simulink model "zaj2simulink"  (R2020b)
settings: Solver=VariableStepAuto  StartTime=0.0  StopTime=100  RelTol=1e-3
settings Model: Creator=bilin  LastModifiedBy=bilin

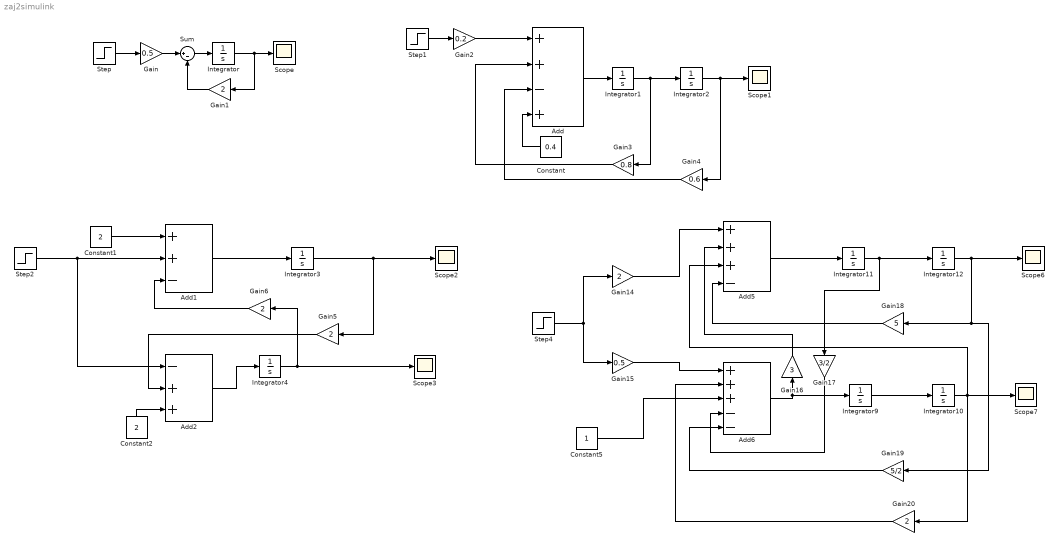
== system zaj2simulink ==
  Add : Sum  Inputs=++-+
  Add1 : Sum  Inputs=++-
  Add2 : Sum  Inputs=-++
  Add5 : Sum  Inputs=+++-
  Add6 : Sum  Inputs=+++--
  Constant : Constant  Value=0.4
  Constant1 : Constant  Value=2
  Constant2 : Constant  Value=2
  Constant5 : Constant
  Gain : Gain  Gain=0.5
  Gain{1,5..6,14,20} (5 alike) : Gain  Gain=2
  Gain15 : Gain  Gain=0.5
  Gain16 : Gain  Gain=3
  Gain17 : Gain  Gain=3/2
  Gain18 : Gain  Gain=5
  Gain19 : Gain  Gain=5/2
  Gain2 : Gain  Gain=0.2
  Gain3 : Gain  Gain=0.8
  Gain4 : Gain  Gain=0.6
  Integrator{,1..4,9..12} (9 alike) : Integrator
  Scope{,1..3,6..7} (6 alike) : Scope
  Step{,1..2,4} (4 alike) : Step  Time=10  After=5  SampleTime=0
  Sum : Sum  Inputs=|+-
  wires:
  Step/1 -> Gain/1
  Gain/1 -> Sum/1
  Sum/1 -> Integrator/1
  Integrator/1 -> Scope/1, Gain1/1
  Gain1/1 -> Sum/2
  Step1/1 -> Gain2/1
  Gain2/1 -> Add/1
  Add/1 -> Integrator1/1
  Constant/1 -> Add/4
  Integrator1/1 -> Integrator2/1, Gain3/1
  Integrator2/1 -> Scope1/1, Gain4/1
  Gain3/1 -> Add/2
  Gain4/1 -> Add/3
  Constant1/1 -> Add1/1
  Step2/1 -> Add2/1, Add1/2
  Add1/1 -> Integrator3/1
  Integrator3/1 -> Gain5/1, Scope2/1
  Constant2/1 -> Add2/3
  Add2/1 -> Integrator4/1
  Integrator4/1 -> Gain6/1, Scope3/1
  Gain6/1 -> Add1/3
  Gain5/1 -> Add2/2
  Step4/1 -> Gain15/1, Gain14/1
  Gain14/1 -> Add5/1
  Gain15/1 -> Add6/1
  Add6/1 -> Integrator9/1, Gain16/1
  Gain16/1 -> Add5/2
  Integrator9/1 -> Integrator10/1
  Add5/1 -> Integrator11/1
  Integrator11/1 -> Gain17/1, Integrator12/1
  Integrator12/1 -> Scope6/1, Gain19/1, Gain18/1
  Gain18/1 -> Add5/4
  Gain17/1 -> Add6/4
  Gain19/1 -> Add6/5
  Constant5/1 -> Add6/3
  Integrator10/1 -> Add5/3, Gain20/1, Scope7/1
  Gain20/1 -> Add6/2
